simulink model "Robot3GDL_Control_Final"  (R2025b)
settings: Solver=VariableStepAuto  StartTime=0.0  StopTime=10.0  RelTol=1e-3
values from neighbouring files (symbols this model uses):
  q0_ic = qd(1,:)' + deg2rad([8; -6; 5])    [crear_modelo_simulink_robot3gdl.m]    (also in robot3dof_TFinal_v2_simulink_generador.m)
  qdot0_ic = [0;0;0]    [crear_modelo_simulink_robot3gdl.m]    (also in robot3dof_TFinal_v2_simulink_generador.m)
  tau_max = [80; 80; 60]    [crear_modelo_simulink_robot3gdl.m]    (also in robot3dof_TFinal_v2_simulink_generador.m)
undefined symbols (not defined in the file or in its folder): gains_ct, gains_pd, gains_pid
settings Model: Creator=OS  LastModifiedBy=OS

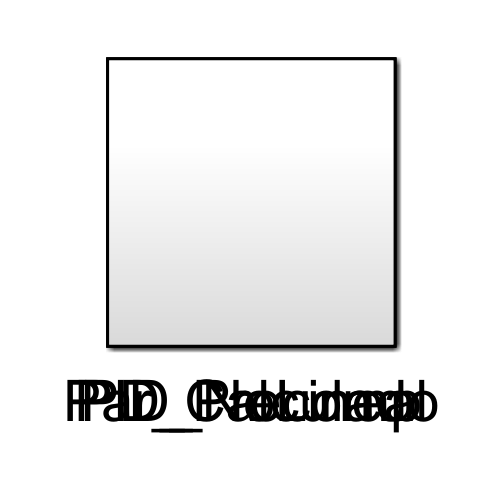
[thumbnail: Simulink's stored preview of the top-level diagram]
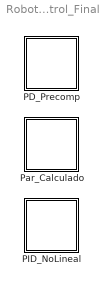
== system Robot3GDL_Control_Final ==
  PD_Precomp : Subsystem
  PID_NoLineal : Subsystem
  Par_Calculado : Subsystem

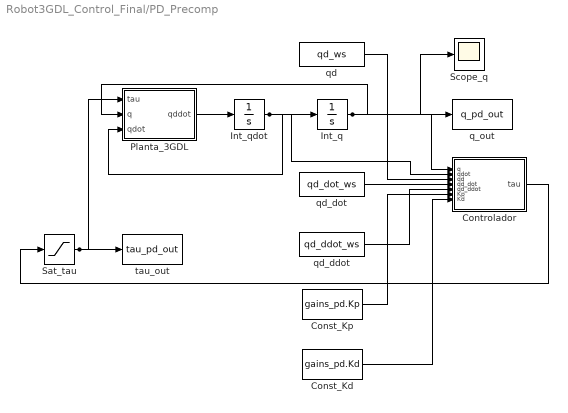
== system Robot3GDL_Control_Final/PD_Precomp ==
  Const_Kd : Constant  Value=gains_pd.Kd
  Const_Kp : Constant  Value=gains_pd.Kp
  Controlador : MATLAB Function  TreatAsAtomicUnit=on
  Int_q : Integrator  InitialCondition=q0_ic
  Int_qdot : Integrator  InitialCondition=qdot0_ic
  Planta_3GDL : MATLAB Function  TreatAsAtomicUnit=on
  Sat_tau : Saturate  UpperLimit=tau_max  LowerLimit=-tau_max
  Scope_q : Scope
  q_out : ToWorkspace  VariableName=q_pd_out  SaveFormat=Timeseries  SampleTime=-1
  qd : FromWorkspace  VariableName=qd_ws
  qd_ddot : FromWorkspace  VariableName=qd_ddot_ws
  qd_dot : FromWorkspace  VariableName=qd_dot_ws
  tau_out : ToWorkspace  VariableName=tau_pd_out  SaveFormat=Timeseries  SampleTime=-1
  wires:
  Planta_3GDL/1(qddot) -> Int_qdot/1
  Sat_tau/1 -> Planta_3GDL/1(tau), tau_out/1
  Const_Kp/1 -> Controlador/6(Kp)
  Int_q/1 -> Planta_3GDL/2(q), q_out/1, Scope_q/1, Controlador/1(q)
  Int_qdot/1 -> Planta_3GDL/3(qdot), Controlador/2(qdot), Int_q/1
  qd_ddot/1 -> Controlador/5(qd_ddot)
  qd_dot/1 -> Controlador/4(qd_dot)
  qd/1 -> Controlador/3(qd)
  Const_Kd/1 -> Controlador/7(Kd)
  Controlador/1(tau) -> Sat_tau/1

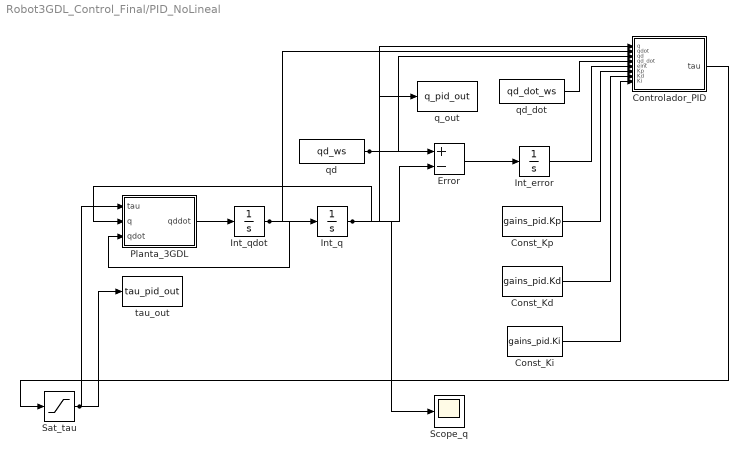
== system Robot3GDL_Control_Final/PID_NoLineal ==
  Const_Kd : Constant  Value=gains_pid.Kd
  Const_Ki : Constant  Value=gains_pid.Ki
  Const_Kp : Constant  Value=gains_pid.Kp
  Controlador_PID : MATLAB Function  TreatAsAtomicUnit=on
  Error : Sum  Inputs=+-
  Int_error : Integrator
  Int_q : Integrator  InitialCondition=q0_ic
  Int_qdot : Integrator  InitialCondition=qdot0_ic
  Planta_3GDL : MATLAB Function  TreatAsAtomicUnit=on
  Sat_tau : Saturate  UpperLimit=tau_max  LowerLimit=-tau_max
  Scope_q : Scope
  q_out : ToWorkspace  VariableName=q_pid_out  SaveFormat=Timeseries  SampleTime=-1
  qd : FromWorkspace  VariableName=qd_ws
  qd_dot : FromWorkspace  VariableName=qd_dot_ws
  tau_out : ToWorkspace  VariableName=tau_pid_out  SaveFormat=Timeseries  SampleTime=-1
  wires:
  Error/1 -> Int_error/1
  Int_qdot/1 -> Planta_3GDL/3(qdot), Controlador_PID/2(qdot), Int_q/1
  Sat_tau/1 -> Planta_3GDL/1(tau), tau_out/1
  Planta_3GDL/1(qddot) -> Int_qdot/1
  qd/1 -> Error/1, Controlador_PID/3(qd)
  Int_q/1 -> Planta_3GDL/2(q), Error/2, q_out/1, Controlador_PID/1(q), Scope_q/1
  Int_error/1 -> Controlador_PID/5(eint)
  qd_dot/1 -> Controlador_PID/4(qd_dot)
  Const_Kp/1 -> Controlador_PID/6(Kp)
  Const_Kd/1 -> Controlador_PID/7(Kd)
  Const_Ki/1 -> Controlador_PID/8(Ki)
  Controlador_PID/1(tau) -> Sat_tau/1

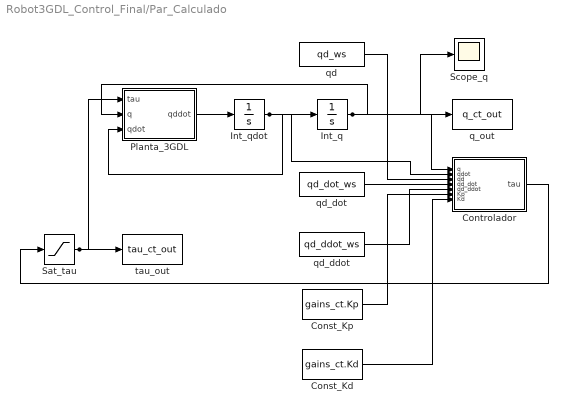
== system Robot3GDL_Control_Final/Par_Calculado ==
  Const_Kd : Constant  Value=gains_ct.Kd
  Const_Kp : Constant  Value=gains_ct.Kp
  Controlador : MATLAB Function  TreatAsAtomicUnit=on
  Int_q : Integrator  InitialCondition=q0_ic
  Int_qdot : Integrator  InitialCondition=qdot0_ic
  Planta_3GDL : MATLAB Function  TreatAsAtomicUnit=on
  Sat_tau : Saturate  UpperLimit=tau_max  LowerLimit=-tau_max
  Scope_q : Scope
  q_out : ToWorkspace  VariableName=q_ct_out  SaveFormat=Timeseries  SampleTime=-1
  qd : FromWorkspace  VariableName=qd_ws
  qd_ddot : FromWorkspace  VariableName=qd_ddot_ws
  qd_dot : FromWorkspace  VariableName=qd_dot_ws
  tau_out : ToWorkspace  VariableName=tau_ct_out  SaveFormat=Timeseries  SampleTime=-1
  wires:
  Sat_tau/1 -> Planta_3GDL/1(tau), tau_out/1
  Const_Kp/1 -> Controlador/6(Kp)
  Int_q/1 -> Planta_3GDL/2(q), Controlador/1(q), Scope_q/1, q_out/1
  Int_qdot/1 -> Planta_3GDL/3(qdot), Controlador/2(qdot), Int_q/1
  Planta_3GDL/1(qddot) -> Int_qdot/1
  Controlador/1(tau) -> Sat_tau/1
  qd_ddot/1 -> Controlador/5(qd_ddot)
  qd_dot/1 -> Controlador/4(qd_dot)
  qd/1 -> Controlador/3(qd)
  Const_Kd/1 -> Controlador/7(Kd)

== matlab function Robot3GDL_Control_Final/PID_NoLineal/Planta_3GDL ==
  data: tau input; qddot output; q input; qdot input
%% BLOQUE MATLAB FUNCTION: Planta Dinamica Robot 3GDL
% Entrada  : tau (3x1), q (3x1), qdot (3x1)
% Salida   : qddot (3x1)
% Pegar el CUERPO de esta funcion dentro del bloque MATLAB Function
% llamado "Planta_3GDL" (ver guia_armado_simulink_robot3gdl.md).
%%

function qddot = mlfb_planta_3gdl(tau, q, qdot)
    % Parametros del robot (identicos a robot3dof_TFinal_v2_dinamica_jacobianos.m)
    L1=0.15; L2=0.5; L3=0.5;
    m1=0.5; m2=0.5; m3=0.5;
    lc1=0.075; lc2=0.25; lc3=0.25;
    g=9.81;
    I1 = diag([0.00105, 0.000225, 0.00105]);
    I2 = diag([0.000225, 0.0105292, 0.0105292]);
    I3 = diag([0.000225, 0.0105292, 0.0105292]);

    M = local_inertia_matrix(q, L1,L2,L3,lc1,lc2,lc3,m1,m2,m3,I1,I2,I3);
    C = local_coriolis_matrix(q, qdot, L1,L2,L3,lc1,lc2,lc3,m1,m2,m3,I1,I2,I3);
    G = local_gravity_vector(q, L2,lc2,lc3,m2,m3,g);
    qddot = M \ (tau - C*qdot - G);
end

function M = local_inertia_matrix(q, L1,L2,L3,lc1,lc2,lc3,m1,m2,m3,I1,I2,I3) %#ok<INUSL>
    q1=q(1); q2=q(2); q3=q(3);
    C1=cos(q1); S1=sin(q1); C2=cos(q2); S2=sin(q2); C23=cos(q2+q3); S23=sin(q2+q3);
    R1 = [C1,0,S1; S1,0,-C1; 0,1,0];
    R2 = [C1*C2,-C1*S2,S1; S1*C2,-S1*S2,-C1; S2,C2,0];
    R3 = [C1*C23,-C1*S23,S1; S1*C23,-S1*S23,-C1; S23,C23,0];
    z0=[0;0;1]; zj=[S1;-C1;0];
    Jv1 = zeros(3,3);
    Jv2 = [-lc2*S1*C2,-lc2*C1*S2,0; lc2*C1*C2,-lc2*S1*S2,0; 0,lc2*C2,0];
    Jv3 = [-S1*(L2*C2+lc3*C23),-C1*(L2*S2+lc3*S23),-C1*lc3*S23; C1*(L2*C2+lc3*C23),-S1*(L2*S2+lc3*S23),-S1*lc3*S23; 0,L2*C2+lc3*C23,lc3*C23];
    Jw1 = [z0,[0;0;0],[0;0;0]];
    Jw2 = [z0,zj,[0;0;0]];
    Jw3 = [z0,zj,zj];
    M = m1*(Jv1.'*Jv1) + Jw1.'*R1*I1*R1.'*Jw1 + ...
        m2*(Jv2.'*Jv2) + Jw2.'*R2*I2*R2.'*Jw2 + ...
        m3*(Jv3.'*Jv3) + Jw3.'*R3*I3*R3.'*Jw3;
    M = (M + M.')/2;
end

function C = local_coriolis_matrix(q, qdot, L1,L2,L3,lc1,lc2,lc3,m1,m2,m3,I1,I2,I3)
    n = 3; h = 1e-6; dM = cell(1,n);
    for k = 1:n
        dq = zeros(n,1); dq(k) = h;
        Mp = local_inertia_matrix(q+dq, L1,L2,L3,lc1,lc2,lc3,m1,m2,m3,I1,I2,I3);
        Mm = local_inertia_matrix(q-dq, L1,L2,L3,lc1,lc2,lc3,m1,m2,m3,I1,I2,I3);
        dM{k} = (Mp - Mm)/(2*h);
    end
    C = zeros(n,n);
    for i=1:n
        for j=1:n
            for k=1:n
                cijk = 0.5*(dM{k}(i,j) + dM{j}(i,k) - dM{i}(j,k));
                C(i,j) = C(i,j) + cijk*qdot(k);
            end
        end
    end
end

function G = local_gravity_vector(q, L2,lc2,lc3,m2,m3,g)
    q2=q(2); q3=q(3);
    G1 = 0;
    G2 = (m2*lc2 + m3*L2)*g*cos(q2) + m3*lc3*g*cos(q2+q3);
    G3 = m3*lc3*g*cos(q2+q3);
    G = [G1; G2; G3];
end

== matlab function Robot3GDL_Control_Final/PID_NoLineal/Controlador_PID ==
  data: q input; tau output; qdot input; qd input; qd_dot input; eint input; Kp input; Kd input; Ki input
%% BLOQUE MATLAB FUNCTION: Control PID no lineal
% Entrada : q, qdot, qd, qd_dot, eint (todos 3x1), Kp,Kd,Ki (3x3 diag)
% Salida  : tau (3x1)
% eint (integral del error) se calcula con un bloque Integrator de
% Simulink ANTES de este bloque, no dentro de el (ver guia).

function tau = mlfb_pid_nolineal(q, qdot, qd, qd_dot, eint, Kp, Kd, Ki)
    % Parametros de gravedad (identicos a robot3dof_TFinal_v2_dinamica_jacobianos.m)
    L2 = 0.5; lc2 = 0.25; lc3 = 0.25; m2 = 0.5; m3 = 0.5; g = 9.81;
    e = qd - q;
    edot = qd_dot - qdot;
    q2 = q(2); q3 = q(3);
    G1 = 0;
    G2 = (m2*lc2 + m3*L2)*g*cos(q2) + m3*lc3*g*cos(q2+q3);
    G3 = m3*lc3*g*cos(q2+q3);
    G = [G1; G2; G3];
    tau = Kp*e + Kd*edot + Ki*eint + G;
end

== matlab function Robot3GDL_Control_Final/PD_Precomp/Controlador ==
  data: q input; tau output; qdot input; qd input; qd_dot input; qd_ddot input; Kp input; Kd input
%% BLOQUE MATLAB FUNCTION: Control PD con precompensacion
% Entrada : q, qdot, qd, qd_dot, qd_ddot (3x1), Kp,Kd (3x3 diag)
% Salida  : tau (3x1)

function tau = mlfb_pd_precomp(q, qdot, qd, qd_dot, qd_ddot, Kp, Kd)
    % Parametros del robot (identicos a robot3dof_TFinal_v2_dinamica_jacobianos.m)
    L1=0.15; L2=0.5; L3=0.5;
    m1=0.5; m2=0.5; m3=0.5;
    lc1=0.075; lc2=0.25; lc3=0.25;
    g=9.81;
    I1 = diag([0.00105, 0.000225, 0.00105]);
    I2 = diag([0.000225, 0.0105292, 0.0105292]);
    I3 = diag([0.000225, 0.0105292, 0.0105292]);

    e = qd - q;
    edot = qd_dot - qdot;
    Mqd = local_inertia_matrix(qd, L1,L2,L3,lc1,lc2,lc3,m1,m2,m3,I1,I2,I3);
    Cqd = local_coriolis_matrix(qd, qd_dot, L1,L2,L3,lc1,lc2,lc3,m1,m2,m3,I1,I2,I3);
    Gqd = local_gravity_vector(qd, L2,lc2,lc3,m2,m3,g);
    tau_ff = Mqd*qd_ddot + Cqd*qd_dot + Gqd;
    tau = tau_ff + Kp*e + Kd*edot;
end

function M = local_inertia_matrix(q, L1,L2,L3,lc1,lc2,lc3,m1,m2,m3,I1,I2,I3) %#ok<INUSL>
    q1=q(1); q2=q(2); q3=q(3);
    C1=cos(q1); S1=sin(q1); C2=cos(q2); S2=sin(q2); C23=cos(q2+q3); S23=sin(q2+q3);
    R1 = [C1,0,S1; S1,0,-C1; 0,1,0];
    R2 = [C1*C2,-C1*S2,S1; S1*C2,-S1*S2,-C1; S2,C2,0];
    R3 = [C1*C23,-C1*S23,S1; S1*C23,-S1*S23,-C1; S23,C23,0];
    z0=[0;0;1]; zj=[S1;-C1;0];
    Jv1 = zeros(3,3);
    Jv2 = [-lc2*S1*C2,-lc2*C1*S2,0; lc2*C1*C2,-lc2*S1*S2,0; 0,lc2*C2,0];
    Jv3 = [-S1*(L2*C2+lc3*C23),-C1*(L2*S2+lc3*S23),-C1*lc3*S23; C1*(L2*C2+lc3*C23),-S1*(L2*S2+lc3*S23),-S1*lc3*S23; 0,L2*C2+lc3*C23,lc3*C23];
    Jw1 = [z0,[0;0;0],[0;0;0]];
    Jw2 = [z0,zj,[0;0;0]];
    Jw3 = [z0,zj,zj];
    M = m1*(Jv1.'*Jv1) + Jw1.'*R1*I1*R1.'*Jw1 + ...
        m2*(Jv2.'*Jv2) + Jw2.'*R2*I2*R2.'*Jw2 + ...
        m3*(Jv3.'*Jv3) + Jw3.'*R3*I3*R3.'*Jw3;
    M = (M + M.')/2;
end

function C = local_coriolis_matrix(q, qdot, L1,L2,L3,lc1,lc2,lc3,m1,m2,m3,I1,I2,I3)
    n = 3; h = 1e-6; dM = cell(1,n);
    for k = 1:n
        dq = zeros(n,1); dq(k) = h;
        Mp = local_inertia_matrix(q+dq, L1,L2,L3,lc1,lc2,lc3,m1,m2,m3,I1,I2,I3);
        Mm = local_inertia_matrix(q-dq, L1,L2,L3,lc1,lc2,lc3,m1,m2,m3,I1,I2,I3);
        dM{k} = (Mp - Mm)/(2*h);
    end
    C = zeros(n,n);
    for i=1:n
        for j=1:n
            for k=1:n
                cijk = 0.5*(dM{k}(i,j) + dM{j}(i,k) - dM{i}(j,k));
                C(i,j) = C(i,j) + cijk*qdot(k);
            end
        end
    end
end

function G = local_gravity_vector(q, L2,lc2,lc3,m2,m3,g)
    q2=q(2); q3=q(3);
    G1 = 0;
    G2 = (m2*lc2 + m3*L2)*g*cos(q2) + m3*lc3*g*cos(q2+q3);
    G3 = m3*lc3*g*cos(q2+q3);
    G = [G1; G2; G3];
end

== matlab function Robot3GDL_Control_Final/PD_Precomp/Planta_3GDL ==
  data: tau input; qddot output; q input; qdot input
%% BLOQUE MATLAB FUNCTION: Planta Dinamica Robot 3GDL
% Entrada  : tau (3x1), q (3x1), qdot (3x1)
% Salida   : qddot (3x1)
% Pegar el CUERPO de esta funcion dentro del bloque MATLAB Function
% llamado "Planta_3GDL" (ver guia_armado_simulink_robot3gdl.md).
%%

function qddot = mlfb_planta_3gdl(tau, q, qdot)
    % Parametros del robot (identicos a robot3dof_TFinal_v2_dinamica_jacobianos.m)
    L1=0.15; L2=0.5; L3=0.5;
    m1=0.5; m2=0.5; m3=0.5;
    lc1=0.075; lc2=0.25; lc3=0.25;
    g=9.81;
    I1 = diag([0.00105, 0.000225, 0.00105]);
    I2 = diag([0.000225, 0.0105292, 0.0105292]);
    I3 = diag([0.000225, 0.0105292, 0.0105292]);

    M = local_inertia_matrix(q, L1,L2,L3,lc1,lc2,lc3,m1,m2,m3,I1,I2,I3);
    C = local_coriolis_matrix(q, qdot, L1,L2,L3,lc1,lc2,lc3,m1,m2,m3,I1,I2,I3);
    G = local_gravity_vector(q, L2,lc2,lc3,m2,m3,g);
    qddot = M \ (tau - C*qdot - G);
end

function M = local_inertia_matrix(q, L1,L2,L3,lc1,lc2,lc3,m1,m2,m3,I1,I2,I3) %#ok<INUSL>
    q1=q(1); q2=q(2); q3=q(3);
    C1=cos(q1); S1=sin(q1); C2=cos(q2); S2=sin(q2); C23=cos(q2+q3); S23=sin(q2+q3);
    R1 = [C1,0,S1; S1,0,-C1; 0,1,0];
    R2 = [C1*C2,-C1*S2,S1; S1*C2,-S1*S2,-C1; S2,C2,0];
    R3 = [C1*C23,-C1*S23,S1; S1*C23,-S1*S23,-C1; S23,C23,0];
    z0=[0;0;1]; zj=[S1;-C1;0];
    Jv1 = zeros(3,3);
    Jv2 = [-lc2*S1*C2,-lc2*C1*S2,0; lc2*C1*C2,-lc2*S1*S2,0; 0,lc2*C2,0];
    Jv3 = [-S1*(L2*C2+lc3*C23),-C1*(L2*S2+lc3*S23),-C1*lc3*S23; C1*(L2*C2+lc3*C23),-S1*(L2*S2+lc3*S23),-S1*lc3*S23; 0,L2*C2+lc3*C23,lc3*C23];
    Jw1 = [z0,[0;0;0],[0;0;0]];
    Jw2 = [z0,zj,[0;0;0]];
    Jw3 = [z0,zj,zj];
    M = m1*(Jv1.'*Jv1) + Jw1.'*R1*I1*R1.'*Jw1 + ...
        m2*(Jv2.'*Jv2) + Jw2.'*R2*I2*R2.'*Jw2 + ...
        m3*(Jv3.'*Jv3) + Jw3.'*R3*I3*R3.'*Jw3;
    M = (M + M.')/2;
end

function C = local_coriolis_matrix(q, qdot, L1,L2,L3,lc1,lc2,lc3,m1,m2,m3,I1,I2,I3)
    n = 3; h = 1e-6; dM = cell(1,n);
    for k = 1:n
        dq = zeros(n,1); dq(k) = h;
        Mp = local_inertia_matrix(q+dq, L1,L2,L3,lc1,lc2,lc3,m1,m2,m3,I1,I2,I3);
        Mm = local_inertia_matrix(q-dq, L1,L2,L3,lc1,lc2,lc3,m1,m2,m3,I1,I2,I3);
        dM{k} = (Mp - Mm)/(2*h);
    end
    C = zeros(n,n);
    for i=1:n
        for j=1:n
            for k=1:n
                cijk = 0.5*(dM{k}(i,j) + dM{j}(i,k) - dM{i}(j,k));
                C(i,j) = C(i,j) + cijk*qdot(k);
            end
        end
    end
end

function G = local_gravity_vector(q, L2,lc2,lc3,m2,m3,g)
    q2=q(2); q3=q(3);
    G1 = 0;
    G2 = (m2*lc2 + m3*L2)*g*cos(q2) + m3*lc3*g*cos(q2+q3);
    G3 = m3*lc3*g*cos(q2+q3);
    G = [G1; G2; G3];
end

== matlab function Robot3GDL_Control_Final/Par_Calculado/Controlador ==
  data: q input; tau output; qdot input; qd input; qd_dot input; qd_ddot input; Kp input; Kd input
%% BLOQUE MATLAB FUNCTION: Control por par calculado
% Entrada : q, qdot, qd, qd_dot, qd_ddot (3x1), Kp,Kd (3x3 diag)
% Salida  : tau (3x1)

function tau = mlfb_par_calculado(q, qdot, qd, qd_dot, qd_ddot, Kp, Kd)
    % Parametros del robot (identicos a robot3dof_TFinal_v2_dinamica_jacobianos.m)
    L1=0.15; L2=0.5; L3=0.5;
    m1=0.5; m2=0.5; m3=0.5;
    lc1=0.075; lc2=0.25; lc3=0.25;
    g=9.81;
    I1 = diag([0.00105, 0.000225, 0.00105]);
    I2 = diag([0.000225, 0.0105292, 0.0105292]);
    I3 = diag([0.000225, 0.0105292, 0.0105292]);

    e = qd - q;
    edot = qd_dot - qdot;
    Mq = local_inertia_matrix(q, L1,L2,L3,lc1,lc2,lc3,m1,m2,m3,I1,I2,I3);
    Cq = local_coriolis_matrix(q, qdot, L1,L2,L3,lc1,lc2,lc3,m1,m2,m3,I1,I2,I3);
    Gq = local_gravity_vector(q, L2,lc2,lc3,m2,m3,g);
    v = qd_ddot + Kd*edot + Kp*e;
    tau = Mq*v + Cq*qdot + Gq;
end

function M = local_inertia_matrix(q, L1,L2,L3,lc1,lc2,lc3,m1,m2,m3,I1,I2,I3) %#ok<INUSL>
    q1=q(1); q2=q(2); q3=q(3);
    C1=cos(q1); S1=sin(q1); C2=cos(q2); S2=sin(q2); C23=cos(q2+q3); S23=sin(q2+q3);
    R1 = [C1,0,S1; S1,0,-C1; 0,1,0];
    R2 = [C1*C2,-C1*S2,S1; S1*C2,-S1*S2,-C1; S2,C2,0];
    R3 = [C1*C23,-C1*S23,S1; S1*C23,-S1*S23,-C1; S23,C23,0];
    z0=[0;0;1]; zj=[S1;-C1;0];
    Jv1 = zeros(3,3);
    Jv2 = [-lc2*S1*C2,-lc2*C1*S2,0; lc2*C1*C2,-lc2*S1*S2,0; 0,lc2*C2,0];
    Jv3 = [-S1*(L2*C2+lc3*C23),-C1*(L2*S2+lc3*S23),-C1*lc3*S23; C1*(L2*C2+lc3*C23),-S1*(L2*S2+lc3*S23),-S1*lc3*S23; 0,L2*C2+lc3*C23,lc3*C23];
    Jw1 = [z0,[0;0;0],[0;0;0]];
    Jw2 = [z0,zj,[0;0;0]];
    Jw3 = [z0,zj,zj];
    M = m1*(Jv1.'*Jv1) + Jw1.'*R1*I1*R1.'*Jw1 + ...
        m2*(Jv2.'*Jv2) + Jw2.'*R2*I2*R2.'*Jw2 + ...
        m3*(Jv3.'*Jv3) + Jw3.'*R3*I3*R3.'*Jw3;
    M = (M + M.')/2;
end

function C = local_coriolis_matrix(q, qdot, L1,L2,L3,lc1,lc2,lc3,m1,m2,m3,I1,I2,I3)
    n = 3; h = 1e-6; dM = cell(1,n);
    for k = 1:n
        dq = zeros(n,1); dq(k) = h;
        Mp = local_inertia_matrix(q+dq, L1,L2,L3,lc1,lc2,lc3,m1,m2,m3,I1,I2,I3);
        Mm = local_inertia_matrix(q-dq, L1,L2,L3,lc1,lc2,lc3,m1,m2,m3,I1,I2,I3);
        dM{k} = (Mp - Mm)/(2*h);
    end
    C = zeros(n,n);
    for i=1:n
        for j=1:n
            for k=1:n
                cijk = 0.5*(dM{k}(i,j) + dM{j}(i,k) - dM{i}(j,k));
                C(i,j) = C(i,j) + cijk*qdot(k);
            end
        end
    end
end

function G = local_gravity_vector(q, L2,lc2,lc3,m2,m3,g)
    q2=q(2); q3=q(3);
    G1 = 0;
    G2 = (m2*lc2 + m3*L2)*g*cos(q2) + m3*lc3*g*cos(q2+q3);
    G3 = m3*lc3*g*cos(q2+q3);
    G = [G1; G2; G3];
end

== matlab function Robot3GDL_Control_Final/Par_Calculado/Planta_3GDL ==
  data: tau input; qddot output; q input; qdot input
%% BLOQUE MATLAB FUNCTION: Planta Dinamica Robot 3GDL
% Entrada  : tau (3x1), q (3x1), qdot (3x1)
% Salida   : qddot (3x1)
% Pegar el CUERPO de esta funcion dentro del bloque MATLAB Function
% llamado "Planta_3GDL" (ver guia_armado_simulink_robot3gdl.md).
%%

function qddot = mlfb_planta_3gdl(tau, q, qdot)
    % Parametros del robot (identicos a robot3dof_TFinal_v2_dinamica_jacobianos.m)
    L1=0.15; L2=0.5; L3=0.5;
    m1=0.5; m2=0.5; m3=0.5;
    lc1=0.075; lc2=0.25; lc3=0.25;
    g=9.81;
    I1 = diag([0.00105, 0.000225, 0.00105]);
    I2 = diag([0.000225, 0.0105292, 0.0105292]);
    I3 = diag([0.000225, 0.0105292, 0.0105292]);

    M = local_inertia_matrix(q, L1,L2,L3,lc1,lc2,lc3,m1,m2,m3,I1,I2,I3);
    C = local_coriolis_matrix(q, qdot, L1,L2,L3,lc1,lc2,lc3,m1,m2,m3,I1,I2,I3);
    G = local_gravity_vector(q, L2,lc2,lc3,m2,m3,g);
    qddot = M \ (tau - C*qdot - G);
end

function M = local_inertia_matrix(q, L1,L2,L3,lc1,lc2,lc3,m1,m2,m3,I1,I2,I3) %#ok<INUSL>
    q1=q(1); q2=q(2); q3=q(3);
    C1=cos(q1); S1=sin(q1); C2=cos(q2); S2=sin(q2); C23=cos(q2+q3); S23=sin(q2+q3);
    R1 = [C1,0,S1; S1,0,-C1; 0,1,0];
    R2 = [C1*C2,-C1*S2,S1; S1*C2,-S1*S2,-C1; S2,C2,0];
    R3 = [C1*C23,-C1*S23,S1; S1*C23,-S1*S23,-C1; S23,C23,0];
    z0=[0;0;1]; zj=[S1;-C1;0];
    Jv1 = zeros(3,3);
    Jv2 = [-lc2*S1*C2,-lc2*C1*S2,0; lc2*C1*C2,-lc2*S1*S2,0; 0,lc2*C2,0];
    Jv3 = [-S1*(L2*C2+lc3*C23),-C1*(L2*S2+lc3*S23),-C1*lc3*S23; C1*(L2*C2+lc3*C23),-S1*(L2*S2+lc3*S23),-S1*lc3*S23; 0,L2*C2+lc3*C23,lc3*C23];
    Jw1 = [z0,[0;0;0],[0;0;0]];
    Jw2 = [z0,zj,[0;0;0]];
    Jw3 = [z0,zj,zj];
    M = m1*(Jv1.'*Jv1) + Jw1.'*R1*I1*R1.'*Jw1 + ...
        m2*(Jv2.'*Jv2) + Jw2.'*R2*I2*R2.'*Jw2 + ...
        m3*(Jv3.'*Jv3) + Jw3.'*R3*I3*R3.'*Jw3;
    M = (M + M.')/2;
end

function C = local_coriolis_matrix(q, qdot, L1,L2,L3,lc1,lc2,lc3,m1,m2,m3,I1,I2,I3)
    n = 3; h = 1e-6; dM = cell(1,n);
    for k = 1:n
        dq = zeros(n,1); dq(k) = h;
        Mp = local_inertia_matrix(q+dq, L1,L2,L3,lc1,lc2,lc3,m1,m2,m3,I1,I2,I3);
        Mm = local_inertia_matrix(q-dq, L1,L2,L3,lc1,lc2,lc3,m1,m2,m3,I1,I2,I3);
        dM{k} = (Mp - Mm)/(2*h);
    end
    C = zeros(n,n);
    for i=1:n
        for j=1:n
            for k=1:n
                cijk = 0.5*(dM{k}(i,j) + dM{j}(i,k) - dM{i}(j,k));
                C(i,j) = C(i,j) + cijk*qdot(k);
            end
        end
    end
end

function G = local_gravity_vector(q, L2,lc2,lc3,m2,m3,g)
    q2=q(2); q3=q(3);
    G1 = 0;
    G2 = (m2*lc2 + m3*L2)*g*cos(q2) + m3*lc3*g*cos(q2+q3);
    G3 = m3*lc3*g*cos(q2+q3);
    G = [G1; G2; G3];
end
